simulink model "VSC_Phase_Shift_AVG_w_Grid"  (R2017b)
settings: Solver=VariableStepAuto  StartTime=0.0  StopTime=sim_time  FixedStep=1e-5  MaxStep=1e-5  RelTol=5e-3  EnableMultiTasking=on
undefined symbols (not defined in the file): cur_sat, f_grid, Gain_p, Kp_is, Kp_pll, L_grid, Ls, omega, P_ref, phase_shift, phase_shift_time, R_grid, Rs, Ti_is, Ti_p, Ti_pll, Vdc, Vs
libraries: powerlib x11, powerlib_extras x1
settings Model: Creator=sigurdjs  LastModifiedBy=Sigurd
settings SolverCC: MaxConsecutiveMinStep=10  ZeroCrossAlgorithm=Adaptive
settings CodeAppCC: StateflowObjectComments=on
settings SimscapeCC: SimscapeNormalizeSystem=off

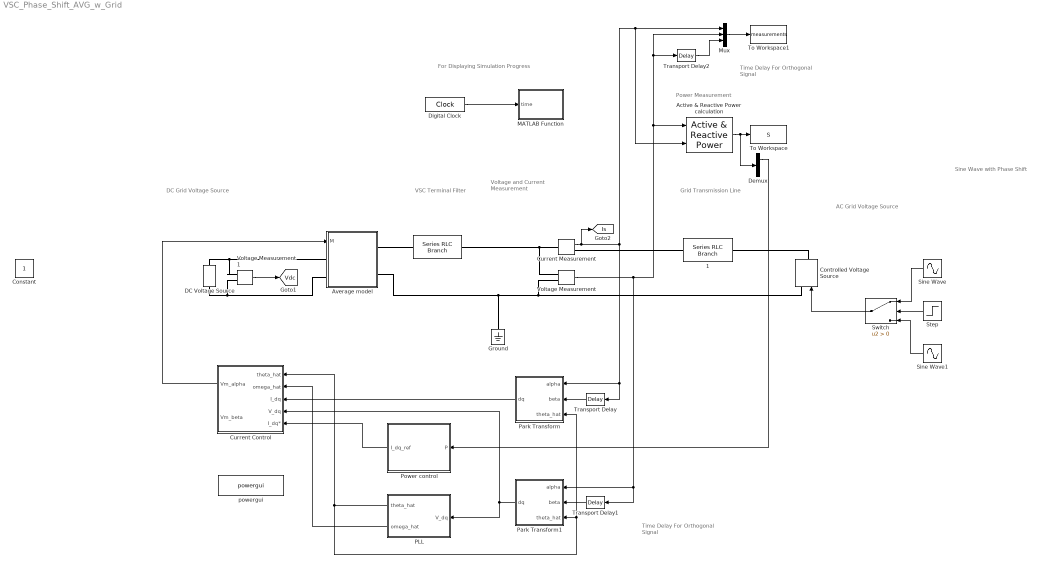
== system VSC_Phase_Shift_AVG_w_Grid ==
  note: For Displaying Simulation Progress
  note: DC Grid
      | Voltage Source
  note: Power Measurement
  note: Time Delay For
      | Orthogonal Signal
  note: VSC Terminal
      | Filter
  note: Voltage and
      | Current Measurement
  note: Time Delay For
      | Orthogonal Signal
  note: Grid Transmission
      | Line
  note: Sine Wave with
      | Phase Shift
  note: AC Grid
      | Voltage Source
  " " : powerlib/Elements/Series RLC Branch  LConnTagsString=__new0  RConnTagsString=__new0  BranchType=RL  Resistance=Rs  Inductance=Ls  SetiL0=off  InitialCurrent=13  Capacitance=1e-6  Setx0=off  InitialVoltage=0  Measurements=None
  " 1" : powerlib/Elements/Series RLC Branch  LConnTagsString=__new0  RConnTagsString=__new0  BranchType=RL  Resistance=R_grid  Inductance=L_grid  SetiL0=off  InitialCurrent=13  Capacitance=1e-6  Setx0=off  InitialVoltage=0  Measurements=None
  Active & Reactive Power calculation : powerlib_extras/Measurements/Active & Reactive Power  f1=f_grid
  Average model : Subsystem
  Controlled Voltage Source : powerlib/Electrical Sources/Controlled Voltage Source  Initialize=off  Source_Type=AC  Amplitude=0  Phase=0  Frequency=0  Measurements=None
  Current Control : Subsystem
  Current Measurement : powerlib/Measurements/Current Measurement  PhasorSimulation=off  OutputType=Complex  PSBequivalent=0
  DC Voltage Source : powerlib/Electrical Sources/DC Voltage Source  Amplitude=Vdc  Measurements=None
  Demux : Demux  Outputs=2
  Digital Clock : DigitalClock  SampleTime=0.01
  Ground : powerlib/Elements/Ground  LConnTagsString=a
  MATLAB Function : MATLAB Function  TreatAsAtomicUnit=on
  Mux : Mux  Inputs=3
  PLL : Subsystem
  Park Transform : Subsystem
  Park Transform1 : Subsystem
  Power control : Subsystem
  Sine Wave : Sin  Amplitude=Vs  Frequency=omega  Phase=phase_shift  SampleTime=0
  Sine Wave1 : Sin  Amplitude=Vs  Frequency=omega  SampleTime=0
  Step : Step  Time=phase_shift_time  SampleTime=0
  Switch : Switch  Criteria=u2 > Threshold
  To Workspace : ToWorkspace  VariableName=S  SaveFormat=Timeseries  SampleTime=-1
  To Workspace1 : ToWorkspace  VariableName=measurements  SaveFormat=Timeseries  SampleTime=-1
  Transport Delay : TransportDelay  DelayTime=1/(4*f_grid)
  Transport Delay1 : TransportDelay  DelayTime=1/(4*f_grid)
  Transport Delay2 : TransportDelay  DelayTime=1/(4*f_grid)
  Voltage Measurement : powerlib/Measurements/Voltage Measurement  PhasorSimulation=off  OutputType=Complex  PSBequivalent=0
  Voltage Measurement1 : powerlib/Measurements/Voltage Measurement  PhasorSimulation=off  OutputType=Complex  PSBequivalent=0
  powergui : powerlib/powergui  Priority=1  SimulationMode=Continuous  SampleTime=1e-5  frequency=60  Iterations=50  frequencyindice=0  Pbase=100e6  ErrMax=1e-4  UnitsV=kV  UnitsW=MW  buscounter=0  FunctionMessages=off  echomessages=off  EnableUseOfTLC=off  CurrentSourceSwitches=off  DisableSnubberDevices=off  DisableRonSwitches=off  DisableVfSwitches=off  DisplayEquations=off  SolverType=Tustin/Backward Euler (TBE)  Interpol=off  ExternalGateDelay=off  methode=off  Ts=100  x0status=blocks  SPID=on  SwTol=0  HookPort=off  RestoreLinks=warning  ResistiveCurrentMeasurement=off  Frange=[0:2:500]  Ylog=off  Xlog=on  ShowGrid=off  save=off  variable=ZData  structure=sps1phPWM1_str1  ZoomFFT=off  StartTime=0.0  cycles=1  DisplayStyle=1  fundamental=100  FreqAxis=off  MaxFrequency=1000  frequencyindicesteady=1  RmsSteady=1  display=off
  Constant : Constant  IOType=siggen
  tag scope: Is=global, Vdc=global
  wires:
  Voltage Measurement/1 -> Park Transform1/1(alpha), Transport Delay1/1, Mux/2, Transport Delay2/1, Active & Reactive Power calculation/1
  PLL/1(theta_hat) -> Current Control/1(theta_hat), Park Transform1/3(theta_hat), Park Transform/3(theta_hat)
  PLL/2(omega_hat) -> Current Control/2(omega_hat)
  Park Transform/1("dq ") -> Current Control/3(I_dq)
  Active & Reactive Power calculation/1 -> Demux/1, To Workspace/1
  Transport Delay/1 -> Park Transform/2(beta)
  Transport Delay1/1 -> Park Transform1/2(beta)
  Park Transform1/1("dq ") -> PLL/1(V_dq), Current Control/4(V_dq)
  Power control/1(I_dq_ref) -> Current Control/5(I_dq*)
  Current Measurement/1 -> Active & Reactive Power calculation/2, Mux/1, Park Transform/1(alpha), Transport Delay/1, [Is]
  Voltage Measurement1/1 -> [Vdc]
  Digital Clock/1 -> MATLAB Function/1(time)
  Mux/1 -> To Workspace1/1
  Transport Delay2/1 -> Mux/3
  Demux/1 -> Power control/1(P)
  Sine Wave1/1 -> Switch/3
  Step/1 -> Switch/2
  Sine Wave/1 -> Switch/1
  Switch/1 -> Controlled Voltage Source/1
  Current Control/1(Vm_alpha) -> Average model/1(M)
  connections:
  Voltage Measurement1/LConn1 -- Average model/LConn1 -- DC Voltage Source/RConn1
  DC Voltage Source/LConn1 -- Average model/LConn2 -- Voltage Measurement1/LConn2
  Voltage Measurement/LConn2 -- Controlled Voltage Source/LConn1 -- Average model/RConn2 -- Ground/LConn1
  Average model/RConn1 -- " "/LConn1
  " "/RConn1 -- Voltage Measurement/LConn1 -- Current Measurement/LConn1
  Controlled Voltage Source/RConn1 -- " 1"/RConn1
  Current Measurement/RConn1 -- " 1"/LConn1

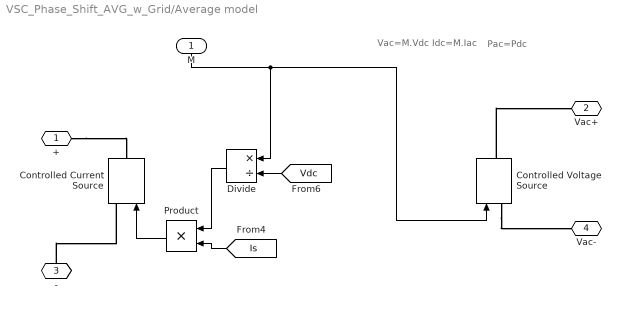
== system VSC_Phase_Shift_AVG_w_Grid/Average model ==
  note: Pac=Pdc
  note: Vac=M.Vdc
      | Idc=M.Iac
  M : Inport
  Controlled Current Source : powerlib/Electrical Sources/Controlled Current Source  Initialize=off  Source_Type=AC  Amplitude=13  Phase=0  Frequency=60  Measurements=None
  Controlled Voltage Source : powerlib/Electrical Sources/Controlled Voltage Source  Initialize=off  Source_Type=AC  Amplitude=120  Phase=90  Frequency=60  Measurements=None
  Divide : Product  Inputs=*/
  Product : Product  RndMeth=Zero
  + : PMIOPort  Port=1  Side=Left
  Vac+ : PMIOPort  Port=2  Side=Right
  - : PMIOPort  Port=3  Side=Left
  Vac- : PMIOPort  Port=4  Side=Right
  wires:
  [Is] -> Product/2
  M/1 -> Divide/1, Controlled Voltage Source/1
  [Vdc] -> Divide/2
  Product/1 -> Controlled Current Source/1
  Divide/1 -> Product/1
  connections:
  Controlled Voltage Source/LConn1 -- Vac-/RConn1
  Controlled Voltage Source/RConn1 -- Vac+/RConn1
  -/RConn1 -- Controlled Current Source/LConn1
  +/RConn1 -- Controlled Current Source/RConn1

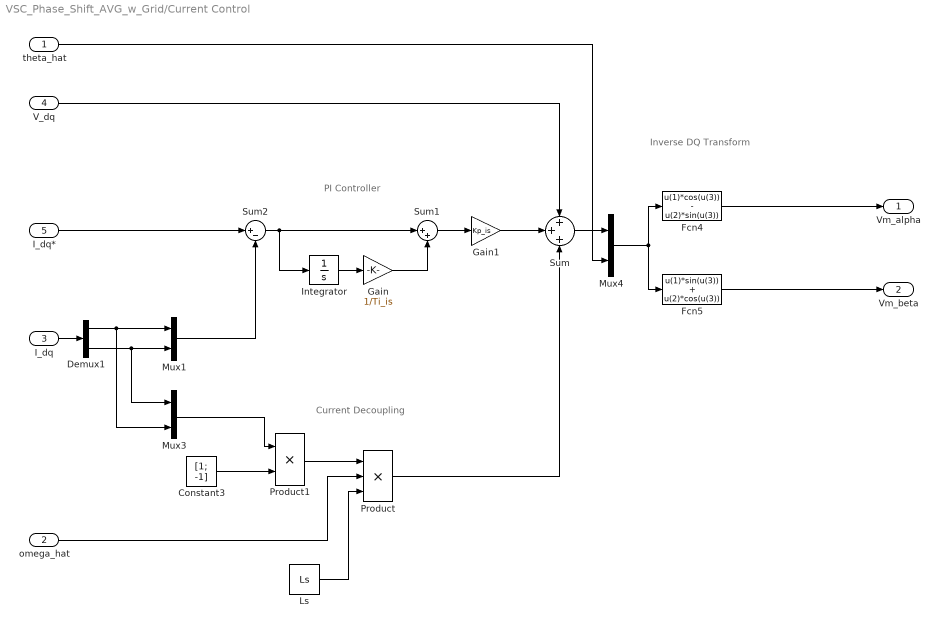
== system VSC_Phase_Shift_AVG_w_Grid/Current Control ==
  note: Inverse
      | DQ Transform
  note: PI Controller
  note: Current Decoupling
  theta_hat : Inport
  omega_hat : Inport  Port=2
  I_dq : Inport  Port=3
  V_dq : Inport  Port=4
  I_dq* : Inport  Port=5
  Constant3 : Constant  Value=[1; -1]
  Demux1 : Demux  Outputs=2
  Fcn4 : Fcn  Expr=u(1)*cos(u(3)) - u(2)*sin(u(3))
  Fcn5 : Fcn  Expr=u(1)*sin(u(3)) + u(2)*cos(u(3))
  Gain : Gain  Gain=1/Ti_is
  Gain1 : Gain  Gain=Kp_is
  Integrator : Integrator
  Ls : Constant  Value=Ls
  Mux1 : Mux  Inputs=2
  Mux3 : Mux  Inputs=2
  Mux4 : Mux  Inputs=2
  Product : Product  Inputs=3
  Product1 : Product
  Sum : Sum  Inputs=+++
  Sum1 : Sum  Inputs=|++
  Sum2 : Sum  Inputs=|+-
  Vm_alpha : Outport
  Vm_beta : Outport  Port=2
  wires:
  Sum2/1 -> Integrator/1, Sum1/1
  Gain1/1 -> Sum/2
  I_dq*/1 -> Sum2/1
  omega_hat/1 -> Product/2
  Mux1/1 -> Sum2/2
  Gain/1 -> Sum1/2
  Ls/1 -> Product/3
  Product1/1 -> Product/1
  theta_hat/1 -> Mux4/2
  Product/1 -> Sum/3
  Integrator/1 -> Gain/1
  Sum1/1 -> Gain1/1
  Constant3/1 -> Product1/2
  I_dq/1 -> Demux1/1
  Demux1/2 -> Mux3/1, Mux1/2
  Mux3/1 -> Product1/1
  Sum/1 -> Mux4/1
  Mux4/1 -> Fcn5/1, Fcn4/1
  Fcn5/1 -> Vm_beta/1
  V_dq/1 -> Sum/1
  Demux1/1 -> Mux1/1, Mux3/2
  Fcn4/1 -> Vm_alpha/1

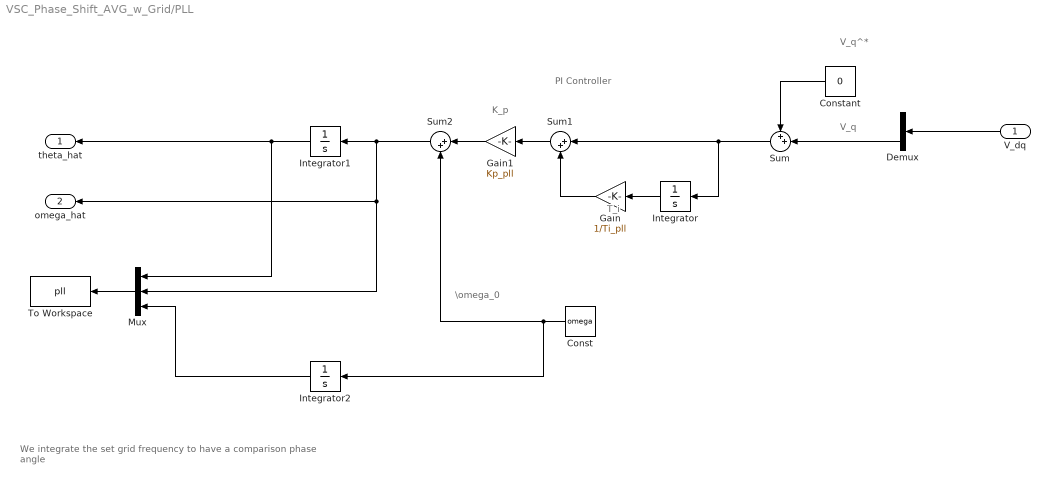
== system VSC_Phase_Shift_AVG_w_Grid/PLL ==
  note: T_i
  note: K_p
  note: \omega_0
  note: V_q
  note: PI Controller
  note: V_q^*
  note: We integrate the set grid frequency to have
      | a comparison phase angle
  V_dq : Inport
  "Const " : Constant  Value=omega
  Constant : Constant  Value=0
  Demux : Demux  Outputs=2
  Gain : Gain  Gain=1/Ti_pll
  Gain1 : Gain  Gain=Kp_pll
  Integrator : Integrator
  Integrator1 : Integrator
  Integrator2 : Integrator
  Mux : Mux  Inputs=3
  Sum : Sum  Inputs=++|
  Sum1 : Sum  Inputs=|++
  Sum2 : Sum  Inputs=|++
  To Workspace : ToWorkspace  VariableName=pll  SaveFormat=Timeseries  SampleTime=-1
  theta_hat : Outport
  omega_hat : Outport  Port=2
  wires:
  Sum1/1 -> Gain1/1
  Integrator/1 -> Gain/1
  Constant/1 -> Sum/1
  Mux/1 -> To Workspace/1
  Gain/1 -> Sum1/2
  Sum2/1 -> Integrator1/1, Mux/2, omega_hat/1
  Gain1/1 -> Sum2/1
  Sum/1 -> Sum1/1, Integrator/1
  Demux/2 -> Sum/2
  V_dq/1 -> Demux/1
  Integrator1/1 -> Mux/1, theta_hat/1
  "Const "/1 -> Sum2/2, Integrator2/1
  Integrator2/1 -> Mux/3

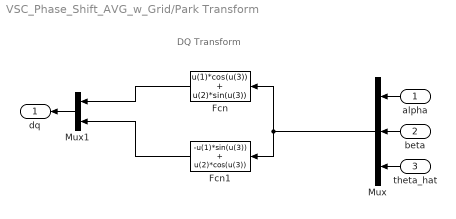
== system VSC_Phase_Shift_AVG_w_Grid/Park Transform ==
  note: DQ Transform
  alpha : Inport
  beta : Inport  Port=2
  theta_hat : Inport  Port=3
  Fcn : Fcn  Expr=u(1)*cos(u(3)) + u(2)*sin(u(3))
  Fcn1 : Fcn  Expr=-u(1)*sin(u(3)) + u(2)*cos(u(3))
  Mux : Mux  Inputs=3
  Mux1 : Mux  Inputs=2
  "dq " : Outport
  wires:
  alpha/1 -> Mux/1
  beta/1 -> Mux/2
  theta_hat/1 -> Mux/3
  Mux/1 -> Fcn1/1, Fcn/1
  Fcn1/1 -> Mux1/2
  Mux1/1 -> "dq "/1
  Fcn/1 -> Mux1/1

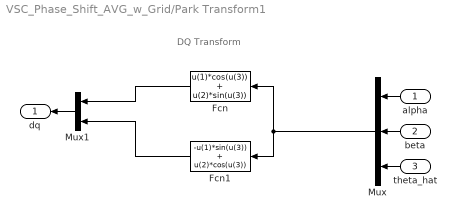
== system VSC_Phase_Shift_AVG_w_Grid/Park Transform1 ==
  note: DQ Transform
  alpha : Inport
  beta : Inport  Port=2
  theta_hat : Inport  Port=3
  Fcn : Fcn  Expr=u(1)*cos(u(3)) + u(2)*sin(u(3))
  Fcn1 : Fcn  Expr=-u(1)*sin(u(3)) + u(2)*cos(u(3))
  Mux : Mux  Inputs=3
  Mux1 : Mux  Inputs=2
  "dq " : Outport
  wires:
  alpha/1 -> Mux/1
  beta/1 -> Mux/2
  theta_hat/1 -> Mux/3
  Mux/1 -> Fcn1/1, Fcn/1
  Fcn1/1 -> Mux1/2
  Mux1/1 -> "dq "/1
  Fcn/1 -> Mux1/1

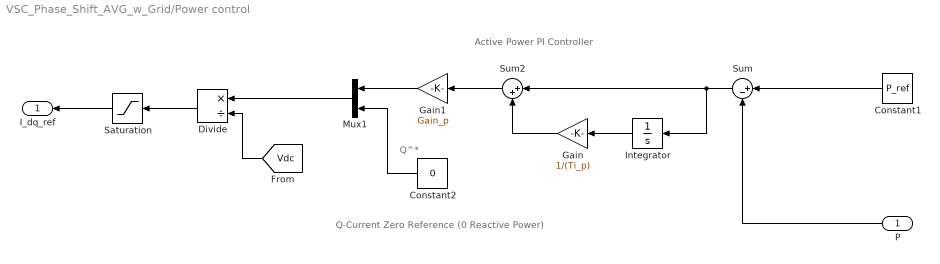
== system VSC_Phase_Shift_AVG_w_Grid/Power control ==
  note: Q^*
  note: Active Power PI Controller
  note: Q-Current Zero Reference
      | (0 Reactive Power)
  P : Inport
  Constant1 : Constant  Value=P_ref
  Constant2 : Constant  Value=0
  Divide : Product  Inputs=*/
  Gain : Gain  Gain=1/(Ti_p)
  Gain1 : Gain  Gain=Gain_p
  Integrator : Integrator
  Mux1 : Mux  Inputs=2
  Saturation : Saturate  UpperLimit=cur_sat  LowerLimit=-cur_sat
  Sum : Sum  Inputs=|+-
  Sum2 : Sum  Inputs=|++
  I_dq_ref : Outport
  wires:
  Gain/1 -> Sum2/2
  Integrator/1 -> Gain/1
  Sum2/1 -> Gain1/1
  Sum/1 -> Integrator/1, Sum2/1
  Gain1/1 -> Mux1/1
  Mux1/1 -> Divide/1
  [Vdc] -> Divide/2
  Saturation/1 -> I_dq_ref/1
  Divide/1 -> Saturation/1
  Constant2/1 -> Mux1/2
  P/1 -> Sum/2
  Constant1/1 -> Sum/1

== matlab function VSC_Phase_Shift_AVG_w_Grid/MATLAB Function ==
  data: time input
function fcn(time)
    fprintf('#######    Simulation currently at %.2f seconds    #######\n', time);
end
